simulink model "Form_Finding_Simulink"  (R2022a)
settings: Solver=ode14x  StartTime=0.0  StopTime=0.1  FixedStep=0.0001  RelTol=1e-3
values from neighbouring files (symbols this model uses):
  a_joint = 160/180*pi    (= 2.79252680319)    [Kinematic_Model_Activation.m]    (also in Kinematic_Model_sweep_double.m; Kinematic_Model_sweep_single.m)
  F_motor = F    (= 50)    [Kinematic_Model_Activation.m]    (also in Kinematic_Model_sweep_double.m; Kinematic_Model_sweep_single.m)
  g = [0;0;-9.81]    [Kinematic_Model_Activation.m]    (also in Kinematic_Model_sweep_double.m; Kinematic_Model_sweep_single.m)
  k_cable = 1200    [Kinematic_Model_Activation.m]    (also in Kinematic_Model_sweep_single.m)
  k_joint = 35    [Kinematic_Model_Activation.m]    (also in Kinematic_Model_sweep_double.m; Kinematic_Model_sweep_single.m)
  l_cable = sqrt(6)/4*l_leg*sin(a_joint/2)*(1 - delta)    [Kinematic_Model_Activation.m]    (also in Kinematic_Model_sweep_double.m; Kinematic_Model_sweep_single.m)
  l_leg = 0.3    [Kinematic_Model_Activation.m]    (also in Kinematic_Model_sweep_double.m; Kinematic_Model_sweep_single.m)
  m_bar = m_leg/2    (= 0.331383847657)    [Kinematic_Model_Activation.m]    (also in Kinematic_Model_sweep_double.m; Kinematic_Model_sweep_single.m)
  x10_ini = N(1:3,10)    [Kinematic_Model_Activation.m]    (also in Kinematic_Model_sweep_double.m; Kinematic_Model_sweep_single.m)
  x11_ini = N(1:3,11)    [Kinematic_Model_Activation.m]    (also in Kinematic_Model_sweep_double.m; Kinematic_Model_sweep_single.m)
  x12_ini = N(1:3,12)    [Kinematic_Model_Activation.m]    (also in Kinematic_Model_sweep_double.m; Kinematic_Model_sweep_single.m)
  x1_ini = N(1:3,1)    [Kinematic_Model_Activation.m]    (also in Kinematic_Model_sweep_double.m; Kinematic_Model_sweep_single.m)
  x2_ini = N(1:3,2)    [Kinematic_Model_Activation.m]    (also in Kinematic_Model_sweep_double.m; Kinematic_Model_sweep_single.m)
  x3_ini = N(1:3,3)    [Kinematic_Model_Activation.m]    (also in Kinematic_Model_sweep_double.m; Kinematic_Model_sweep_single.m)
  x4_ini = N(1:3,4)    [Kinematic_Model_Activation.m]    (also in Kinematic_Model_sweep_double.m; Kinematic_Model_sweep_single.m)
  x5_ini = N(1:3,5)    [Kinematic_Model_Activation.m]    (also in Kinematic_Model_sweep_double.m; Kinematic_Model_sweep_single.m)
  x6_ini = N(1:3,6)    [Kinematic_Model_Activation.m]    (also in Kinematic_Model_sweep_double.m; Kinematic_Model_sweep_single.m)
  x7_ini = N(1:3,7)    [Kinematic_Model_Activation.m]    (also in Kinematic_Model_sweep_double.m; Kinematic_Model_sweep_single.m)
  x8_ini = N(1:3,8)    [Kinematic_Model_Activation.m]    (also in Kinematic_Model_sweep_double.m; Kinematic_Model_sweep_single.m)
  x9_ini = N(1:3,9)    [Kinematic_Model_Activation.m]    (also in Kinematic_Model_sweep_double.m; Kinematic_Model_sweep_single.m)
(part 2 of 2)

== matlab function Form_Finding_Simulink/6 joints/Force bar 5--11 ==
  data: torsion_i output; torsion_j output; xi input; xj input; m input; k_joint input; alpha input; l_bar input; a_joint input; g input
function [torsion_i, torsion_j]= Force(xi, xj, m, k_joint, alpha, l_bar, a_joint,g)
% Node distance
dist = norm(xj-xi);

% Force exerted by the joint at the end node. The force is zero when the
% deflection angle is larger than a_joint
if alpha < a_joint
    F_torsion = 1/2 * k_joint * (a_joint - alpha) / (cos(alpha/2)*l_bar/2);
else
    F_torsion = 0;
end

% Gravity
Fg_j = m*g/2;

% Calculation of the two parts of the torsion
torsion_i = F_torsion *(xi-xj)/dist + Fg_j;
torsion_j = F_torsion *(xj-xi)/dist + Fg_j;

end

== matlab function Form_Finding_Simulink/6 joints/Joint bar 6--12 ==
  data: xi input; alpha output; xj input; xk input; l input; x_joint output
function [alpha, x_joint]  = angle(xi, xj, xk, l)
%% Calculating the angle
d = norm(xi - xj); % Nodal distance
mag = (l^2-2*d^2)/l^2; % Term inside the inverse cosine to calculate the angle
alpha = acos(mag); % Angle of the joint

%% Plotting the Joint
% Distance from axis
d = l/2*cos(alpha/2);

% Vectors used for determination of the normal vector
nxi = transpose(xi);
nxj = transpose(xj);
nxk = transpose(xk);

% Normal vector of a plane created by a set of 2 parallel bars
normal = cross(nxi-nxj, nxi-nxk);
N = normal/norm(normal);

% Vector along the line between bar-connected nodes
x = nxj - nxi;
X = x/norm(x);

% Vector pointing outwards 
V = rotVec(X,N,-90);

% Position vector of the joint, to be used for plotting
x_joint = transpose(d*V + (nxj+nxi)/2);

end

== matlab function Form_Finding_Simulink/24 cables/cable 1--4 ==
  data: out_i output; E_cable output; out_j output; k_cable input; l_cable input; xi input; xj input
function [out_i, E_cable, out_j]= cable(k_cable, l_cable,xi,xj)
% Node distance
dist = norm(xi-xj);

% Difference of node distance with the cable rest length
D = dist-l_cable;

% If the cable is in tension, then the force is calculated. When the cable is slack, the force is zero 
if  dist-l_cable >= 0
    D = dist-l_cable;
elseif dist-l_cable < 0
    D = 0;
end

% Forces on end nodes
out_i = k_cable*D*(xj-xi)/dist;
out_j = -k_cable*D*(xj-xi)/dist;

% Potential energy stored in the cable
E_cable = 0.5*k_cable*D^2;
end

== matlab function Form_Finding_Simulink/6 joints/Force bar 6--12 ==
  data: T input; xi input; xj input; m input; torsion_i output; torsion_j output; k_joint input; alpha input; l_bar input; a_joint input; g input
function [torsion_i, torsion_j]= Force(T, xi, xj, m, k_joint, alpha, l_bar, a_joint, g)
% Node distance
dist = norm(xj-xi);

% Force exerted by the joint at the end node. The force is zero when the
% deflection angle is larger than a_joint
if alpha < a_joint
    F_torsion = 1/2 * k_joint * (a_joint - alpha) / (cos(alpha/2)*l_bar/2);
else
    F_torsion = 0;
end

% Gravitational force:
Fg_j = m*g/2;

% Motor Force, also with the lever effect incorporated
F_motor = T/(l_bar*cos(alpha/2));

% Calculation of the two parts of the torsion
torsion_i = (F_torsion - F_motor) *(xi-xj)/dist; % % No gravity on this node because it is on the ground
torsion_j = (F_torsion - F_motor) *(xj-xi)/dist + Fg_j;

end

== matlab function Form_Finding_Simulink/12 nodes /node  4/MATLAB Function ==
  data: X input; F_out output; F_in input
function F_out = ground_constraint(X,F_in)
if X(3) <= 0 && F_in(3) < 0 
    F_out = [F_in(1);F_in(2);0];
else
    F_out = F_in;
end
end

== matlab function Form_Finding_Simulink/12 nodes /node  7/MATLAB Function ==
  data: X input; F_out output; F_in input
function F_out = ground_constraint(X,F_in)
if X(3) <= 0 && F_in(3) < 0 
    F_out = [F_in(1);F_in(2);0];
else
    F_out = F_in;
end
end

== matlab function Form_Finding_Simulink/12 nodes /node  8/MATLAB Function ==
  data: X input; F_out output; F_in input
function F_out = ground_constraint(X,F_in)
if X(3) <= 0 && F_in(3) < 0 
    F_out = [F_in(1);F_in(2);0];
else
    F_out = F_in;
end

end

== matlab function Form_Finding_Simulink/12 nodes /node  9/MATLAB Function ==
  data: X input; F_out output; F_in input
function F_out = ground_constraint(X,F_in)
if X(3) <= 0 && F_in(3) < 0 
    F_out = [F_in(1);F_in(2);0];
else
    F_out = F_in;
end
end

== matlab function Form_Finding_Simulink/12 nodes /node  10/MATLAB Function ==
  data: X input; F_out output; F_in input
function F_out = ground_constraint(X,F_in)
if X(3) <= 0 && F_in(3) < 0 
    F_out = [F_in(1);F_in(2);0];
else
    F_out = F_in;
end
end

== matlab function Form_Finding_Simulink/12 nodes /node  11/MATLAB Function ==
  data: X input; F_out output; F_in input
function F_out = ground_constraint(X,F_in)
if X(3) <= 0 && F_in(3) < 0 
    F_out = [F_in(1);F_in(2);0];
else
    F_out = F_in;
end
end

== matlab function Form_Finding_Simulink/12 nodes /node  12/MATLAB Function1 ==
  data: X input; F_out output; F_in input
function F_out = ground_constraint(X,F_in)
if X(3) <= 0 && F_in(3) < 0 
    F_out = [F_in(1);F_in(2);0];
else
    F_out = F_in;
end
end

== matlab function Form_Finding_Simulink/24 cables/cable 2--3 ==
  data: out_i output; E_cable output; out_j output; k_cable input; l_cable input; xi input; xj input
function [out_i, E_cable, out_j]= cable(k_cable, l_cable,xi,xj)
% Node distance
dist = norm(xi-xj);

% Difference of node distance with the cable rest length
D = dist-l_cable;

% If the cable is in tension, then the force is calculated. When the cable is slack, the force is zero 
if  dist-l_cable >= 0
    D = dist-l_cable;
elseif dist-l_cable < 0
    D = 0;
end

% Forces on end nodes
out_i = k_cable*D*(xj-xi)/dist;
out_j = -k_cable*D*(xj-xi)/dist;

% Potential energy stored in the cable
E_cable = 0.5*k_cable*D^2;
end

== matlab function Form_Finding_Simulink/12 nodes /node  3/node 1 constrain ==
  data: control_out output; control_in input
function control_out = node3_control(control_in)

control_out = [control_in(1);control_in(2);0];
end

== matlab function Form_Finding_Simulink/12 nodes /node 1/node 1 constrain ==
  data: control_out output; control_in input
function control_out = node1_control(control_in)

control_out = [control_in(1);control_in(2);0];
end

== matlab function Form_Finding_Simulink/6 joints/Jumping direction ==
  data: alpha_p input; l_bar input; xi input; xj input; xk input; xl input; theta output; clearance output
function [theta, clearance] = Jump_Direction(alpha_p, l_bar, xi, xj, xk, xl)
% Transposes
nxi = transpose(xi);
nxj = transpose(xj);
nxk = transpose(xk);
nxl = transpose(xl);

% Normal vector
normal1 = cross(nxi-nxj, nxi-nxk);
normal2 = cross(nxi-nxl, nxi-nxk);

% Normalized
N1 = normal1/norm(normal1);
N2 = normal2/norm(normal2);

% Caclulation of jumping direction
CosTheta = max(min(dot(N2,N1)/(norm(N2)*norm(N1)),1),-1);
theta = real(acos(CosTheta));

% Calculation of lowest joint distance to ground (leg 3)
clearance = l_bar*sin(alpha_p/2 - theta);

end
